simulink model "impulse_response_simulink"  (R2019a)
settings: Solver=VariableStepAuto  StartTime=0.0  StopTime=45  RelTol=1e-3
libraries: dspsrcs4 x1
settings Model: Creator=raxit  LastModifiedBy=raxit

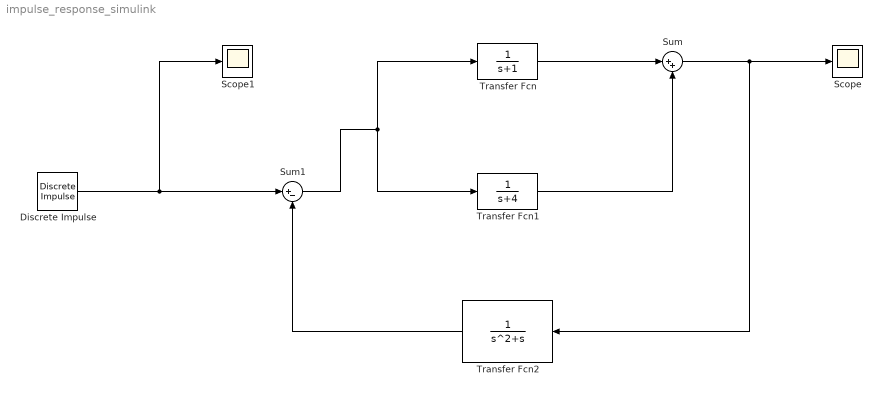
== system impulse_response_simulink ==
  Discrete Impulse : dspsrcs4/Discrete  Impulse  Delay=0  SampleTime=1  FrameSample=1  OutputFrames=off  dataType=double  isSigned=on  wordLen=16  udDataType=sfix(16)  fracBitsMode=Best precision  numFracBits=15  OutDataTypeStr=double  LastOutDataTypeStr=double
  Scope : Scope
  Scope1 : Scope
  Sum : Sum  Inputs=|++
  Sum1 : Sum  Inputs=|+-
  Transfer Fcn : TransferFcn  Denominator=[1 1]
  Transfer Fcn1 : TransferFcn  Denominator=[1 4]
  Transfer Fcn2 : TransferFcn  Denominator=[1 1 0]
  wires:
  Transfer Fcn2/1 -> Sum1/2
  Sum1/1 -> Transfer Fcn1/1, Transfer Fcn/1
  Transfer Fcn/1 -> Sum/1
  Transfer Fcn1/1 -> Sum/2
  Sum/1 -> Transfer Fcn2/1, Scope/1
  Discrete Impulse/1 -> Scope1/1, Sum1/1
